simulink model "MEAS_Speed_Read"  (R2022b)
settings: Solver=FixedStepDiscrete  StartTime=0.0  StopTime=10.0  RelTol=1e-3  EnableMultiTasking=on
InitFcn:
  | mbd_mpc_consistency_checks(bdroot(gcs));
undefined symbols (not defined in the file): AngleChangeDir, I_MAX, LQFP, OffsetSelector, PhA_Offset, PhB_Offset, SpdChangeDir, SpdFilterConst
libraries: mbd_mpc574x_ec_toolbox x18, ammclib_bam_mpc574x x9, simulink x1, mcbpositiondecoderlib x1
settings Model: Creator=MAAM  LastModifiedBy=MAAM
settings DataIOCC: ExternalInput=off  InitialState=off  SaveOutput=off  SignalLogging=off  SaveTime=off
settings OptimizationCC: DefaultParameterBehavior=Inlined  EnhancedBackFolding=on  PassReuseOutputArgsAs=Individual arguments  ZeroExternalMemoryAtStartup=off  ZeroInternalMemoryAtStartup=off  OptimizeBlockOrder=speed  DifferentSizesBufferReuse=on  OptimizationCustomize=off  EfficientTunableParamExpr=on
settings DebuggingCC: InheritedTsInSrcMsg=none  ParameterTunabilityLossMsg=error
settings HardwareCC: ProdBitPerPointer=32  ProdBitPerSizeT=32  ProdBitPerPtrDiffT=32  ProdLargestAtomicInteger=Long  ProdLargestAtomicFloat=Double  ProdEndianess=BigEndian  ProdWordSize=32  ProdHWDeviceType=Motorola PowerPC
settings ModelReferenceCC: ModelReferenceNumInstancesAllowed=Single
settings SFSimCC: MATLABDynamicMemAlloc=off
settings RTWCC: Description=Model Based Design Toolbox MPC57xx Code Generation Target  SystemTargetFile=mbd_mpc574x.tlc  MakeCommand=mbd_mpc574x_make_rtw  TemplateMakefile=mbd_mpc574x.tmf
settings CodeAppCC: ForceParamTrailComments=on  IgnoreCustomStorageClasses=off  OperatorAnnotations=on  SimulinkDataObjDesc=on  SFDataObjDesc=on  InsertBlockDesc=on
settings STFCustomTargetCC: TargetLangStandard=C99 (ISO)  MultiwordLength=256  CombineOutputUpdateFcns=on  ERTCustomFileBanners=on  SupportContinuousTime=off  SupportNonInlinedSFcns=off  RemoveResetFunc=on  MATLABClassNameForMDSCustomization=Simulink.SoftwareTarget.ERTCustomization  SystemTargetFile=mbd_mpc574x.tlc
settings ERTTargetCC: TargetLangStandard=C99 (ISO)  ParMdlRefBuildCompliant=off  CompOptLevelCompliant=off  ConcurrentExecutionCompliant=off  ModelStepFunctionPrototypeControlCompliant=off  CPPClassGenCompliant=off  UseToolchainInfoCompliant=off  InlinedParameterPlacement=NonHierarchical  ERTCustomFileTemplate=example_file_process.tlc

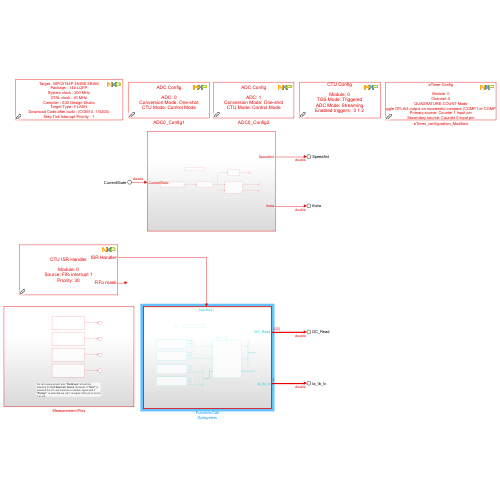
[thumbnail: Simulink's stored preview of the top-level diagram]
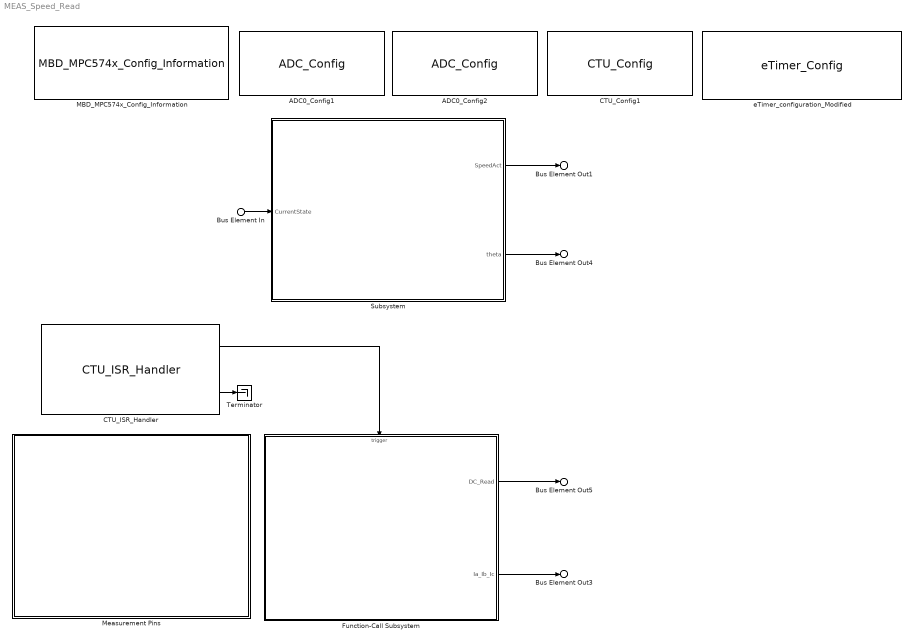
== system MEAS_Speed_Read ==
  Bus Element In : Inport  PortName=CurrentState
  ADC0_Config1 : mbd_mpc574x_ec_toolbox/Motor Control Blocks/ADC Blocks/ADC_Config  Priority=9  adc_instance=0  adc_mode=One-shot  adc_ctu=Control Mode  adc_channels_no_n=3  adc_channel_n_0=PTB9: [ADC0_AN11 | Analog function AN11 of ADC0]  adc_channel_n_1=PTB12: [ADC0_AN14 | Analog function AN14 of ADC0]  adc_channel_n_2=PTB8: [ADC0_AN1 | Analog function AN1 of ADC0]  adc_channel_n_3=not available  adc_channel_n_4=not available  adc_channel_n_5=not available  adc_channel_n_6=not available  adc_channel_n_7=not available  adc_channel_n_8=not available  adc_channel_n_9=not available  adc_channel_n_10=not available  adc_channel_n_11=not available  adc_channel_n_12=not available  adc_channel_n_13=not available  adc_channel_n_14=not available  adc_channel_n_15=not available  adc_channel_n_16=not available  adc_channel_n_17=not available  adc_channel_n_18=not available  adc_channel_n_19=not available  adc_channel_n_20=not available  adc_channel_n_21=not available  adc_channel_n_22=not available  adc_channel_n_23=not available  adc_channel_n_24=not available  adc_channel_n_25=not available  adc_channel_n_26=not available  adc_channel_n_27=not available  adc_channel_n_28=not available  adc_channel_n_29=not available  adc_channel_n_30=not available  adc_channel_n_31=not available  adc_channel_n_32=not available  adc_channel_n_33=not available  adc_channel_n_34=not available  adc_channel_n_35=not available  adc_channel_n_36=not available  adc_channel_n_37=not available  adc_channel_n_38=not available  adc_channel_n_39=not available  adc_channel_n_40=not available  adc_channel_n_41=not available  adc_channel_n_42=not available  adc_channel_n_43=not available  adc_channel_n_44=not available  adc_channel_n_45=not available  adc_channel_n_46=not available  adc_channel_n_47=not available  show_adv_opts=on  adc_prec=8  adc_presample_0=High voltage ground for ADC  adc_int=8  adc_presample_1=High voltage ground for ADC  adc_ext=8  adc_presample_2=High voltage ground for ADC  adc_clk=Equal to bus clock  adc_ack=off  adc_ext_trigger=External Trigger Disabled  adc_skip_sampling=off  adc_calibration=on  adc_wls=Right  adc_owr=off  adc_inj_trigger=Injected Trigger Disabled  adc_mux_delay=0  adc_decode_delay=0  adc_thr_reg_no=0  adc_upper_value_0=0  adc_lower_value_0=0  adc_upper_value_1=0  adc_lower_value_1=0  adc_upper_value_2=0  adc_lower_value_2=0  adc_upper_value_3=0  adc_lower_value_3=0  adc_upper_value_4=0  adc_lower_value_4=0  adc_upper_value_5=0  adc_lower_value_5=0  adc_upper_value_6=0  adc_lower_value_6=0  adc_upper_value_7=0  adc_lower_value_7=0  adc_upper_value_8=0  adc_lower_value_8=0  adc_upper_value_9=0  adc_lower_value_9=0  adc_upper_value_10=0  adc_lower_value_10=0  adc_upper_value_11=0  adc_lower_value_11=0  adc_upper_value_12=0  adc_lower_value_12=0  adc_upper_value_13=0  adc_lower_value_13=0  adc_upper_value_14=0  adc_lower_value_14=0  adc_upper_value_15=0  adc_lower_value_15=0  adc_wdt_isr_init=off  adc_en_wdt_0=off  adc_th_index_0=0  adc_en_wdt_1=off  adc_th_index_1=0  adc_en_wdt_2=off  adc_th_index_2=0  adc_en_wdt_3=off  adc_th_index_3=0  adc_en_wdt_4=off  adc_th_index_4=0  adc_en_wdt_5=off  adc_th_index_5=0  adc_en_wdt_6=off  adc_th_index_6=0  adc_en_wdt_7=off  adc_th_index_7=0  adc_en_wdt_8=off  adc_th_index_8=0  adc_en_wdt_9=off  adc_th_index_9=0  adc_en_wdt_10=off  adc_th_index_10=0  adc_en_wdt_11=off  adc_th_index_11=0  adc_en_wdt_12=off  adc_th_index_12=0  adc_en_wdt_13=off  adc_th_index_13=0  adc_en_wdt_14=off  adc_th_index_14=0  adc_en_wdt_15=off  adc_th_index_15=0  adc_en_wdt_16=off  adc_th_index_16=0  adc_en_wdt_17=off  adc_th_index_17=0  adc_en_wdt_18=off  adc_th_index_18=0  adc_en_wdt_19=off  adc_th_index_19=0  adc_en_wdt_20=off  adc_th_index_20=0  adc_en_wdt_21=off  adc_th_index_21=0  adc_en_wdt_22=off  adc_th_index_22=0  adc_en_wdt_23=off  adc_th_index_23=0  adc_en_wdt_24=off  adc_th_index_24=0  adc_en_wdt_25=off  adc_th_index_25=0  adc_en_wdt_26=off  adc_th_index_26=0  adc_en_wdt_27=off  adc_th_index_27=0  adc_en_wdt_28=off  adc_th_index_28=0  adc_en_wdt_29=off  adc_th_index_29=0  adc_en_wdt_30=off  adc_th_index_30=0  adc_en_wdt_31=off  adc_th_index_31=0  adc_en_wdt_32=off  adc_th_index_32=0  adc_en_wdt_33=off  adc_th_index_33=0  adc_en_wdt_34=off  adc_th_index_34=0  adc_en_wdt_35=off  adc_th_index_35=0  adc_en_wdt_36=off  adc_th_index_36=0  adc_en_wdt_37=off  adc_th_index_37=0  adc_en_wdt_38=off  adc_th_index_38=0  adc_en_wdt_39=off  adc_th_index_39=0  adc_en_wdt_40=off  adc_th_index_40=0  adc_en_wdt_41=off  adc_th_index_41=0  adc_en_wdt_42=off  adc_th_index_42=0  adc_en_wdt_43=off  adc_th_index_43=0  adc_en_wdt_44=off  adc_th_index_44=0  adc_en_wdt_45=off  adc_th_index_45=0  adc_en_wdt_46=off  adc_th_index_46=0  adc_en_wdt_47=off  adc_th_index_47=0
  ADC0_Config2 : mbd_mpc574x_ec_toolbox/Motor Control Blocks/ADC Blocks/ADC_Config  Priority=9  adc_instance=1  adc_mode=One-shot  adc_ctu=Control Mode  adc_channels_no_n=1  adc_channel_n_0=PTB10: [ADC1_AN12 | Analog function AN12 of ADC1]  adc_channel_n_1=not available  adc_channel_n_2=not available  adc_channel_n_3=not available  adc_channel_n_4=not available  adc_channel_n_5=not available  adc_channel_n_6=not available  adc_channel_n_7=not available  adc_channel_n_8=not available  adc_channel_n_9=not available  adc_channel_n_10=not available  adc_channel_n_11=not available  adc_channel_n_12=not available  adc_channel_n_13=not available  adc_channel_n_14=not available  adc_channel_n_15=not available  adc_channel_n_16=not available  adc_channel_n_17=not available  adc_channel_n_18=not available  adc_channel_n_19=not available  adc_channel_n_20=not available  adc_channel_n_21=not available  adc_channel_n_22=not available  adc_channel_n_23=not available  adc_channel_n_24=not available  adc_channel_n_25=not available  adc_channel_n_26=not available  adc_channel_n_27=not available  adc_channel_n_28=not available  adc_channel_n_29=not available  adc_channel_n_30=not available  adc_channel_n_31=not available  adc_channel_n_32=not available  adc_channel_n_33=not available  adc_channel_n_34=not available  adc_channel_n_35=not available  adc_channel_n_36=not available  adc_channel_n_37=not available  adc_channel_n_38=not available  adc_channel_n_39=not available  adc_channel_n_40=not available  adc_channel_n_41=not available  adc_channel_n_42=not available  adc_channel_n_43=not available  adc_channel_n_44=not available  adc_channel_n_45=not available  adc_channel_n_46=not available  adc_channel_n_47=not available  show_adv_opts=on  adc_prec=8  adc_presample_0=High voltage ground for ADC  adc_int=8  adc_presample_1=High voltage ground for ADC  adc_ext=8  adc_presample_2=High voltage ground for ADC  adc_clk=Equal to bus clock  adc_ack=off  adc_ext_trigger=External Trigger Disabled  adc_skip_sampling=off  adc_calibration=on  adc_wls=Right  adc_owr=off  adc_inj_trigger=Injected Trigger Disabled  adc_mux_delay=0  adc_decode_delay=0  adc_thr_reg_no=0  adc_upper_value_0=0  adc_lower_value_0=0  adc_upper_value_1=0  adc_lower_value_1=0  adc_upper_value_2=0  adc_lower_value_2=0  adc_upper_value_3=0  adc_lower_value_3=0  adc_upper_value_4=0  adc_lower_value_4=0  adc_upper_value_5=0  adc_lower_value_5=0  adc_upper_value_6=0  adc_lower_value_6=0  adc_upper_value_7=0  adc_lower_value_7=0  adc_upper_value_8=0  adc_lower_value_8=0  adc_upper_value_9=0  adc_lower_value_9=0  adc_upper_value_10=0  adc_lower_value_10=0  adc_upper_value_11=0  adc_lower_value_11=0  adc_upper_value_12=0  adc_lower_value_12=0  adc_upper_value_13=0  adc_lower_value_13=0  adc_upper_value_14=0  adc_lower_value_14=0  adc_upper_value_15=0  adc_lower_value_15=0  adc_wdt_isr_init=off  adc_en_wdt_0=off  adc_th_index_0=0  adc_en_wdt_1=off  adc_th_index_1=0  adc_en_wdt_2=off  adc_th_index_2=0  adc_en_wdt_3=off  adc_th_index_3=0  adc_en_wdt_4=off  adc_th_index_4=0  adc_en_wdt_5=off  adc_th_index_5=0  adc_en_wdt_6=off  adc_th_index_6=0  adc_en_wdt_7=off  adc_th_index_7=0  adc_en_wdt_8=off  adc_th_index_8=0  adc_en_wdt_9=off  adc_th_index_9=0  adc_en_wdt_10=off  adc_th_index_10=0  adc_en_wdt_11=off  adc_th_index_11=0  adc_en_wdt_12=off  adc_th_index_12=0  adc_en_wdt_13=off  adc_th_index_13=0  adc_en_wdt_14=off  adc_th_index_14=0  adc_en_wdt_15=off  adc_th_index_15=0  adc_en_wdt_16=off  adc_th_index_16=0  adc_en_wdt_17=off  adc_th_index_17=0  adc_en_wdt_18=off  adc_th_index_18=0  adc_en_wdt_19=off  adc_th_index_19=0  adc_en_wdt_20=off  adc_th_index_20=0  adc_en_wdt_21=off  adc_th_index_21=0  adc_en_wdt_22=off  adc_th_index_22=0  adc_en_wdt_23=off  adc_th_index_23=0  adc_en_wdt_24=off  adc_th_index_24=0  adc_en_wdt_25=off  adc_th_index_25=0  adc_en_wdt_26=off  adc_th_index_26=0  adc_en_wdt_27=off  adc_th_index_27=0  adc_en_wdt_28=off  adc_th_index_28=0  adc_en_wdt_29=off  adc_th_index_29=0  adc_en_wdt_30=off  adc_th_index_30=0  adc_en_wdt_31=off  adc_th_index_31=0  adc_en_wdt_32=off  adc_th_index_32=0  adc_en_wdt_33=off  adc_th_index_33=0  adc_en_wdt_34=off  adc_th_index_34=0  adc_en_wdt_35=off  adc_th_index_35=0  adc_en_wdt_36=off  adc_th_index_36=0  adc_en_wdt_37=off  adc_th_index_37=0  adc_en_wdt_38=off  adc_th_index_38=0  adc_en_wdt_39=off  adc_th_index_39=0  adc_en_wdt_40=off  adc_th_index_40=0  adc_en_wdt_41=off  adc_th_index_41=0  adc_en_wdt_42=off  adc_th_index_42=0  adc_en_wdt_43=off  adc_th_index_43=0  adc_en_wdt_44=off  adc_th_index_44=0  adc_en_wdt_45=off  adc_th_index_45=0  adc_en_wdt_46=off  adc_th_index_46=0  adc_en_wdt_47=off  adc_th_index_47=0
  CTU_Config1 : mbd_mpc574x_ec_toolbox/Motor Control Blocks/CTU Blocks/CTU_Config  Priority=10  ctuModule=0  ctuPrescaler=1  ctuTGS=Triggered  ctuTGSCCV=7000  ctuTGSCLM=0  ctuExtMode=Toggle  ctuTGSADC=Streaming  ctuMrsInput=PWM Reload  ctuMrsInputEdge=Rising Edge  ctuMrsIsrEnable=off  ctuIsrErrEnable=off  ctuDMAGREEnable=off  ctuMRSDMAEnable=off  ctuDisableoutput=off  ctuShowAdvOpts=on  inputPwmRel=Rising Edge  inputPwmOdd0=Disabled  inputPwmOdd1=Disabled  inputPwmOdd2=Disabled  inputPwmOdd3=Disabled  inputPwmEven0=Disabled  inputPwmEven1=Disabled  inputPwmEven3=Disabled  inputPwmEven2=Disabled  inputPwmReal0=Disabled  inputPwmReal1=Disabled  inputPwmReal2=Disabled  inputPwmReal3=Disabled  inputeTimer1=Disabled  inputeTimer2=Disabled  inputExternal=Disabled  trgEn0=on  trgEn1=on  trgEn2=on  trgEn3=off  trgEn4=off  trgEn5=off  trgEn6=off  trgEn7=off  trgCmp0=250  trgExt0=off  trgTmr0_0=off  trgTmr1_0=off  trgTmr2_0=off  trgInt0=off  trgAdc0=on  trgAdcStart0=0  trgAdcStop0=0  trgCmp1=1000  trgExt1=off  trgTmr0_1=off  trgTmr1_1=off  trgTmr2_1=off  trgInt1=off  trgAdc1=on  trgAdcStart1=1  trgAdcStop1=1  trgCmp2=0  trgExt2=off  trgTmr0_2=off  trgTmr1_2=off  trgTmr2_2=off  trgInt2=off  trgAdc2=on  trgAdcStart2=2  trgAdcStop2=2  trgCmp3=0  trgExt3=off  trgTmr0_3=off  trgTmr1_3=off  trgTmr2_3=off  trgInt3=off  trgAdc3=off  trgAdcStart3=0  trgAdcStop3=0  trgCmp4=0  trgExt4=off  trgTmr0_4=off  trgTmr1_4=off  trgTmr2_4=off  trgInt4=off  trgAdc4=off  trgAdcStart4=0  trgAdcStop4=0  trgCmp5=0  trgExt5=off  trgTmr0_5=off  trgTmr1_5=off  trgTmr2_5=off  trgAdc5=off  trgInt5=off  trgAdcStart5=0  trgAdcStop5=0  trgCmp6=0  trgExt6=off  trgTmr0_6=off  trgTmr1_6=off  trgTmr2_6=off  trgInt6=off  trgAdc6=off  trgAdcStart6=0  trgAdcStop6=0  trgCmp7=0  trgExt7=off  trgTmr0_7=off  trgTmr1_7=off  trgTmr2_7=off  trgInt7=off  trgAdc7=off  trgAdcStart7=0  trgAdcStop7=0  fifoTh0=1  fifoIsrOVR0=off  fifoIsrOVF0=off  fifoIsrEmpty0=off  fifoIsrFull0=off  fifoDMA0=off  fifoTh1=3  fifoIsrOVR1=off  fifoIsrOVF1=on  fifoIsrEmpty1=off  fifoIsrFull1=off  fifoDMA1=off  fifoTh2=0  fifoIsrOVR2=off  fifoIsrOVF2=off  fifoIsrEmpty2=off  fifoIsrFull2=off  fifoDMA2=off  fifoTh3=0  fifoIsrOVR3=off  fifoIsrOVF3=off  fifoIsrEmpty3=off  fifoIsrFull3=off  fifoDMA3=off  pinInternal=None  pinExternal=PTC14: [CTU0_EXT_TGR | CTU0 External Trigger Output]  ctuAdcCmdNumber=3  adc_ie_0=off  adc_fifo_0=1  adc_conv_mode_0=Single Conversion  adc_port_0=Port A  adc_channel_0=14  adc_channel_a_0=0  adc_channel_b_0=0  adc_ie_1=off  adc_fifo_1=1  adc_conv_mode_1=Single Conversion  adc_port_1=Port A  adc_channel_1=1  adc_channel_a_1=0  adc_channel_b_1=0  adc_ie_2=off  adc_fifo_2=1  adc_conv_mode_2=Dual Conversion  adc_port_2=Port A  adc_channel_2=11  adc_channel_a_2=11  adc_channel_b_2=12  adc_ie_3=off  adc_fifo_3=1  adc_conv_mode_3=Single Conversion  adc_port_3=Port B  adc_channel_3=12  adc_channel_a_3=0  adc_channel_b_3=0  adc_ie_4=off  adc_fifo_4=0  adc_conv_mode_4=Single Conversion  adc_port_4=Port A  adc_channel_4=0  adc_channel_a_4=0  adc_channel_b_4=0  adc_ie_5=off  adc_fifo_5=0  adc_conv_mode_5=Single Conversion  adc_port_5=Port A  adc_channel_5=0  adc_channel_a_5=0  adc_channel_b_5=0  adc_ie_6=off  adc_fifo_6=0  adc_conv_mode_6=Single Conversion  adc_port_6=Port A  adc_channel_6=0  adc_channel_a_6=0  adc_channel_b_6=0  adc_ie_7=off  adc_fifo_7=0  adc_conv_mode_7=Single Conversion  adc_port_7=Port A  adc_channel_7=0  adc_channel_a_7=0  adc_channel_b_7=0  adc_ie_8=off  adc_fifo_8=0  adc_conv_mode_8=Single Conversion  adc_port_8=Port A  adc_channel_8=0  adc_channel_a_8=0  adc_channel_b_8=0  adc_ie_9=off  adc_fifo_9=0  adc_conv_mode_9=Single Conversion  adc_port_9=Port A  adc_channel_9=0  adc_channel_a_9=0  adc_channel_b_9=0  adc_ie_10=off  adc_fifo_10=0  adc_conv_mode_10=Single Conversion  adc_port_10=Port A  adc_channel_10=0  adc_channel_a_10=0  adc_channel_b_10=0  adc_ie_11=off  adc_fifo_11=0  adc_conv_mode_11=Single Conversion  adc_port_11=Port A  adc_channel_11=0  adc_channel_a_11=0  adc_channel_b_11=0  adc_ie_12=off  adc_fifo_12=1  adc_conv_mode_12=Single Conversion  adc_port_12=Port A  adc_channel_12=0  adc_channel_a_12=0  adc_channel_b_12=0  adc_ie_13=off  adc_fifo_13=3  adc_conv_mode_13=Single Conversion  adc_port_13=Port A  adc_channel_13=0  adc_channel_a_13=0  adc_channel_b_13=0  adc_ie_14=off  adc_fifo_14=0  adc_conv_mode_14=Single Conversion  adc_port_14=Port A  adc_channel_14=0  adc_channel_a_14=0  adc_channel_b_14=0  adc_ie_15=off  adc_fifo_15=0  adc_conv_mode_15=Single Conversion  adc_port_15=Port A  adc_channel_15=0  adc_channel_a_15=0  adc_channel_b_15=0  adc_ie_16=off  adc_fifo_16=0  adc_conv_mode_16=Single Conversion  adc_port_16=Port A  adc_channel_16=0  adc_channel_a_16=0  adc_channel_b_16=0  adc_ie_17=off  adc_fifo_17=0  adc_conv_mode_17=Single Conversion  adc_port_17=Port A  adc_channel_17=0  adc_channel_a_17=0  adc_channel_b_17=0  adc_ie_18=off  adc_fifo_18=0  adc_conv_mode_18=Single Conversion  adc_port_18=Port A  adc_channel_18=0  adc_channel_a_18=0  adc_channel_b_18=0  adc_ie_19=off  adc_fifo_19=0  adc_conv_mode_19=Single Conversion  adc_port_19=Port A  adc_channel_19=0  adc_channel_a_19=0  adc_channel_b_19=0  adc_ie_20=off  adc_fifo_20=0  adc_conv_mode_20=Single Conversion  adc_port_20=Port A  adc_channel_20=0  adc_channel_a_20=0  adc_channel_b_20=0  adc_ie_21=off  adc_fifo_21=0  adc_conv_mode_21=Single Conversion  adc_port_21=Port A  adc_channel_21=0  adc_channel_a_21=0  adc_channel_b_21=0  adc_ie_22=off  adc_fifo_22=0  adc_conv_mode_22=Single Conversion  adc_port_22=Port A  adc_channel_22=0  adc_channel_a_22=0  adc_channel_b_22=0  adc_ie_23=off  adc_fifo_23=0  adc_conv_mode_23=Single Conversion  adc_port_23=Port A  adc_channel_23=0  adc_channel_a_23=0  adc_channel_b_23=0
  CTU_ISR_Handler : mbd_mpc574x_ec_toolbox/Motor Control Blocks/CTU Blocks/CTU_ISR_Handler  ctuModule=0  ctuIsrSource=Fifo interrupt  ctuIsrPriority=30  ctuIsrTrigger=1  ctuIsrFifo=1
  Function-Call Subsystem : Subsystem  TreatAsAtomicUnit=on
  MBD_MPC574x_Config_Information : mbd_mpc574x_ec_toolbox/MBD_MPC574x_Config_Information  Priority=1  disp_str=|  config_params=[]  mcu_target_name=MPC5744P  mcu_target_package=144-LQFP  mcu_target_sram_size=384KB  mcu_system_clock_freq=200  mcu_xtal_freq=40  mcu_step_timer=PIT Channel 0  mcu_step_priority=1  ds_import_enable=on  target_compiler=S32 Design Studio  target_memory=FLASH  s32ds_target_compile_opts=-g3 -mbig -mvle -O1 -mregnames -mlsp -specs=ewl_c9x.specs -mhard-float -Wall -c -std=c99 -fdata-sections -ffunction-sections -funsigned-char -fmessage-length=0 -nostdinc -fno-jump-tables -DTURN_ON_CPU0  s32ds_target_assemble_opts=-g3 -mbig -mvle -mregnames -O1 -DTURN_ON_CPU0 -mhard-float  s32ds_target_link_opts=-Xlinker -gc-sections  s32ds_target_default_lcf=on  s32ds_target_user_lcf=MPC5744P_flash.ld  ghs_target_compile_opts=-G -filetype.c  ghs_target_assemble_opts=-G -filetype.assembly  ghs_target_default_lcf=on  ghs_target_user_lcf=MPC5744P_flash.ld  diab_target_compile_opts=-@E+err.log -c -g -Xenum-is-best -Xlint -Xnested-interrupts -Xdebug-local-cie -Xclib-optim-off -Xc-new  diab_target_assemble_opts=-@E+err.log -l -g  diab_target_link_opts=-@E+err.log -Ws -m6 -lc -lm  diab_target_default_lcf=on  diab_target_user_lcf=MPC5744P_flash.dld  pil_download_enable=off  rbl_download_enable=on  rbl_start_delay=5000  rbl_restart_request=on  rbl_com_port=Custom  rbl_com_port_custom=COM10  pil_download_rate=115200  pil_interface=Serial 0  pil_rx=PTB3: [LIN0_RX | LIN 0 Receive Pin]  pil_tx=PTB2: [LIN0_TX | LINFlexD 0 Transmit Pin]  rbl_def_password=on  rbl_password=0xFEEDFACECAFEBEEF  rbl_manual_len_size=off  rbl_start_address=0  rbl_code_size=0  ADC_PcrCheckEnDis=on  FlexPWM_PcrCheckEnDis=on  CTU_PcrCheckEnDis=on  SWG_PcrCheckEnDis=on  eTimer_PcrCheckEnDis=off  EQADC_PcrCheckEnDis=on  eMIOS_PcrCheckEnDis=on  FlexCAN_PcrCheckEnDis=on  I2C_PcrCheckEnDis=on  MCAN_PcrCheckEnDis=on  SPI_PcrCheckEnDis=on  UART_PcrCheckEnDis=on  GPIO_OutputPcrCheckEnDis=on  GPIO_InputPcrCheckEnDis=on  eDMA_PcrCheckEnDis=on  PIT_PcrCheckEnDis=on  AMMCLIB_PcrCheckEnDis=on  FM_PcrCheckEnDis=on  Profiler_PcrCheckEnDis=on  ModelRef_PcrCheckEnDis=on  ModelPinCheck_PcrCheckEnDis=on
      | System Clock : 200 MHz
      | Target : MPC5744P
      | Package : 144LQFP
      | XTAL Freq : 40 MHz
      | Compiler : S32 Design Studio
      | Target Type : FLASH
      | Global Interrupt Priority : 8
      | System Tick Interrupt Priority : 12
      | Freemaster : None;
      | Download Code after build : off
  Measurement Pins : Subsystem
  Subsystem : Subsystem
  Terminator : Terminator
  eTimer_configuration_Modified : mbd_mpc574x_ec_toolbox/Motor Control Blocks/eTIMER Blocks/eTimer_Config  etimerModule=0  etimerChannel=0  etimerMode=QUADRATURE-COUNT Mode  etimerCountOnce=Count repeatedly  etimerCountLength=Count until compare and then reinitialize  etimerCountDirection=Count down  etimerCountStart=on  etimerCaptureArm=on  etimerShowAdv=on  etimerPrimarySource=Counter 1 input pin  etimerPrimaryPolarity=True polarity  etimerSecondarySource=Counter 0 input pin  etimerSecondaryPolarity=True polarity  etimerSampleCount=Require 3 consecutive samples to be of equal value  etimerSamplePeriod=1  etimerOutEnable=The external pin is configured as an input  etimerOutPolarity=True polarity  etimerOutMode=Toggle OFLAG output on successful compare (COMP1 or COMP2)  etimerCompMode=COMP1 is used when the counter is counting up and COMP2 when counting down  etimerCompLoad1=Load CNTR with CMPLD upon successful compare with the value in COMP2  etimerCompLoad2=Load CNTR with CMPLD upon successful compare with the value in COMP1  etimerCapt1=Capture any edge  etimerCapt2=Capture any edge  etimerOneShot=Free running mode is selected  etimerMasterMode=Disable broadcast of this channel output  etimerCoForce=Other channels cannot force this channel output  etimerCoChanInit=Other channels cannot force re-initialization of this channel  etimerRedundant=off  etimerCOMP1init=3999  etimerCOMP2init=0  etimerCNTRinit=0  etimerCh0=PTA0: [eTimer0_ETC0 | eTimer_0 Input Data Channel 0]  etimerCh1=PTA1: [eTimer0_ETC1 | eTimer_0 Input Data Channel 1]  etimerCh2=None  etimerCh3=None  etimerCh4=None  etimerCh5=None  etimerIsrTCFIE=off  etimerIsrTCF1IE=off  etimerIsrTCF2IE=off  etimerIsrTOFIE=off  etimerIsrIELFIE=off  etimerIsrIEHFIE=off  etimerIsrICF1IE=off  etimerIsrICF2IE=off  etimerIsrRCF=off  etimerIsrWDF=off
  Bus Element Out1 : Outport  PortName=SpeedAct
  Bus Element Out3 : Outport  Port=2  PortName=Ia_Ib_Ic
  Bus Element Out4 : Outport  Port=3  PortName=theta
  Bus Element Out5 : Outport  Port=4  PortName=DC_Read
  wires:
  Subsystem/1(SpeedAct) -> Bus Element Out1/1
  CTU_ISR_Handler/2 -> Terminator/1
  CTU_ISR_Handler/1 -> Function-Call Subsystem/Trigger
  Function-Call Subsystem/2(Ia_Ib_Ic) -> Bus Element Out3/1
  Subsystem/2(theta) -> Bus Element Out4/1
  Function-Call Subsystem/1(DC_Read) -> Bus Element Out5/1
  Bus Element In/1 -> Subsystem/1(CurrentState)

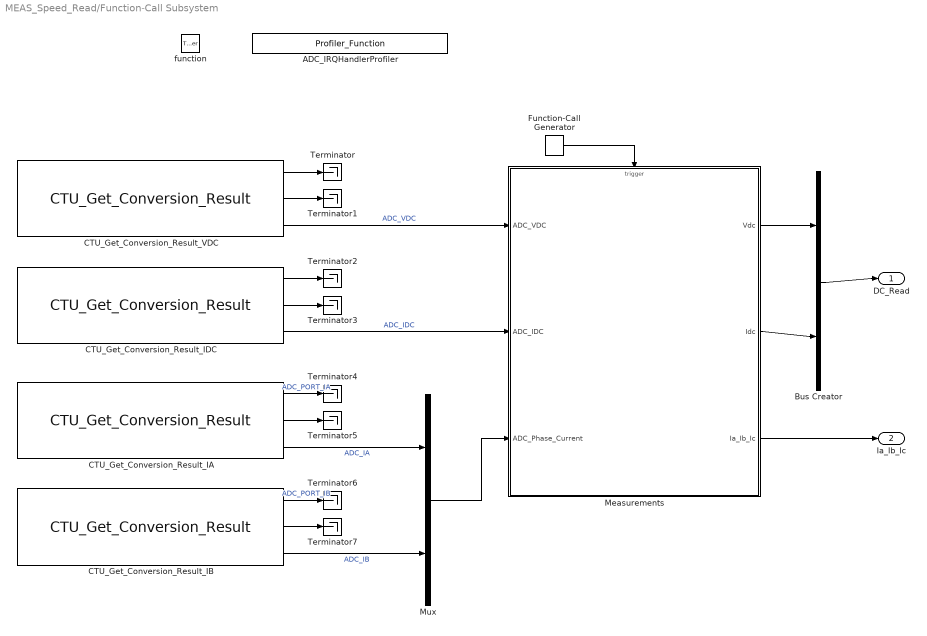
== system MEAS_Speed_Read/Function-Call Subsystem ==
  function : TriggerPort  TriggerType=function-call  VariantControl=(inherit)
  ADC_IRQHandlerProfiler : mbd_mpc574x_ec_toolbox/Utility Blocks/Profiler_Function  profile_index=2
  Bus Creator : BusCreator  Inputs=2
  CTU_Get_Conversion_Result_IA : mbd_mpc574x_ec_toolbox/Motor Control Blocks/CTU Blocks/CTU_Get_Conversion_Result  Priority=3  ctuModule=0  ctuFifoIndex=1  ctuAlign=Right unsigned
  CTU_Get_Conversion_Result_IB : mbd_mpc574x_ec_toolbox/Motor Control Blocks/CTU Blocks/CTU_Get_Conversion_Result  Priority=4  ctuModule=0  ctuFifoIndex=1  ctuAlign=Right unsigned
  CTU_Get_Conversion_Result_IDC : mbd_mpc574x_ec_toolbox/Motor Control Blocks/CTU Blocks/CTU_Get_Conversion_Result  Priority=2  ctuModule=0  ctuFifoIndex=1  ctuAlign=Right unsigned
  CTU_Get_Conversion_Result_VDC : mbd_mpc574x_ec_toolbox/Motor Control Blocks/CTU Blocks/CTU_Get_Conversion_Result  Priority=1  ctuModule=0  ctuFifoIndex=1  ctuAlign=Right unsigned
  Function-Call Generator : simulink/Ports & Subsystems/Function-Call Generator  sample_time=-1  numberOfIterations=1  DisallowWideOutput=off
  Measurements : Subsystem  TreatAsAtomicUnit=on
  Mux : Mux  Inputs=2
  Terminator{,1..7} (8 alike) : Terminator
  DC_Read : Outport
  Ia_Ib_Ic : Outport  Port=2
  wires:
  CTU_Get_Conversion_Result_IB/2 -> Terminator7/1
  CTU_Get_Conversion_Result_IB/1 -> Terminator6/1  "ADC_PORT_IB"
  CTU_Get_Conversion_Result_IA/2 -> Terminator5/1
  CTU_Get_Conversion_Result_IA/1 -> Terminator4/1  "ADC_PORT_IA"
  CTU_Get_Conversion_Result_IDC/2 -> Terminator3/1
  CTU_Get_Conversion_Result_IDC/1 -> Terminator2/1
  CTU_Get_Conversion_Result_VDC/2 -> Terminator1/1
  CTU_Get_Conversion_Result_VDC/1 -> Terminator/1
  CTU_Get_Conversion_Result_IB/3 -> Mux/2  "ADC_IB"
  CTU_Get_Conversion_Result_IA/3 -> Mux/1  "ADC_IA"
  Mux/1 -> Measurements/3(ADC_Phase_Current)
  Function-Call Generator/1 -> Measurements/Trigger
  CTU_Get_Conversion_Result_IDC/3 -> Measurements/2(ADC_IDC)  "ADC_IDC"
  CTU_Get_Conversion_Result_VDC/3 -> Measurements/1(ADC_VDC)  "ADC_VDC"
  Measurements/1(Vdc) -> Bus Creator/1
  Measurements/2(Idc) -> Bus Creator/2
  Measurements/3(Ia_Ib_Ic) -> Ia_Ib_Ic/1
  Bus Creator/1 -> DC_Read/1

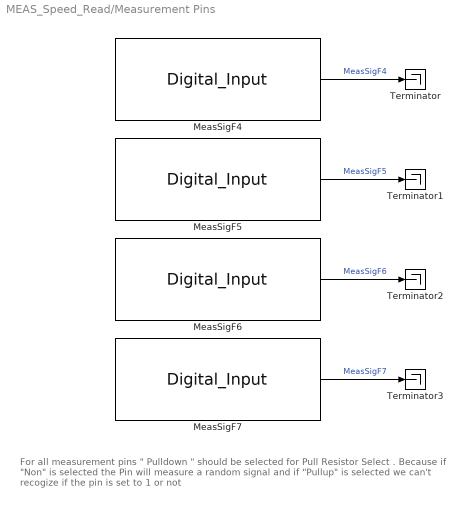
== system MEAS_Speed_Read/Measurement Pins ==
  note: For all measurement pins " Pulldown " should be selected for Pull Resistor Select . Because if "Non" is selected the Pin will measure a random signal and if "Pullup" is selected we can't recogize if the pin is set to 1 or not
  MeasSigF4 : mbd_mpc574x_ec_toolbox/GPIO Blocks/Digital_Input  gpio_pin=PTF4: [SIUL2_GPIO84 | General Purpose IO PF[4]]  pull_resistor=Pulldown
  MeasSigF5 : mbd_mpc574x_ec_toolbox/GPIO Blocks/Digital_Input  gpio_pin=PTF5: [SIUL2_GPIO85 | General Purpose IO PF[5]]  pull_resistor=Pulldown
  MeasSigF6 : mbd_mpc574x_ec_toolbox/GPIO Blocks/Digital_Input  gpio_pin=PTF6: [SIUL2_GPIO86 | General Purpose IO PF[6]]  pull_resistor=Pulldown
  MeasSigF7 : mbd_mpc574x_ec_toolbox/GPIO Blocks/Digital_Input  gpio_pin=PTE7: [SIUL2_GPI71 | General Purpose IO PE[7]]  pull_resistor=Pulldown
  Terminator{,1..3} (4 alike) : Terminator
  wires:
  MeasSigF5/1 -> Terminator1/1  "MeasSigF5"
  MeasSigF4/1 -> Terminator/1  "MeasSigF4"
  MeasSigF7/1 -> Terminator3/1  "MeasSigF7"
  MeasSigF6/1 -> Terminator2/1  "MeasSigF6"

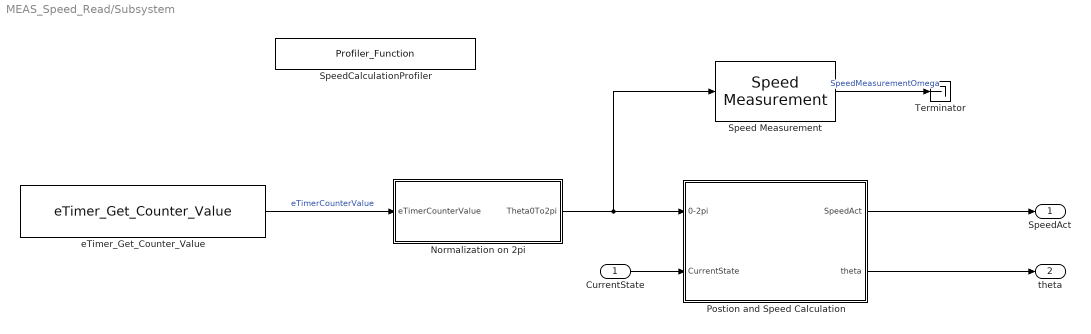
== system MEAS_Speed_Read/Subsystem ==
  CurrentState : Inport
  Normalization on 2pi : Subsystem
  Postion and Speed Calculation : Subsystem
  Speed Measurement : mcbpositiondecoderlib/Speed Measurement  PositionUnit=Radians  PositionScalingDatatype=uint32  SpeedCalculationMode=Maximum application speed  SampleTimeAsync=100e-6  MaximumApplicationSpeed=3000  SpeedResolution=5e-6  DelayLength=99  MaximumMeasurableSpeed=3000  MeasurableSpeedResolution=1.397e-06  SpeedUnit=RPM  PerUnitSpeed=1000  SpeedDataType=single
  "SpeedCalculationProfiler   " : mbd_mpc574x_ec_toolbox/Utility Blocks/Profiler_Function  profile_index=4
  Terminator : Terminator
  eTimer_Get_Counter_Value : mbd_mpc574x_ec_toolbox/Motor Control Blocks/eTIMER Blocks/eTimer_Get_Counter_Value  etimerModule=0  etimerChannel=0
  SpeedAct : Outport
  theta : Outport  Port=2
  wires:
  Normalization on 2pi/1(Theta0To2pi) -> Speed Measurement/1, Postion and Speed Calculation/1(0-2pi)
  Speed Measurement/1 -> Terminator/1  "SpeedMeasurementOmega"
  eTimer_Get_Counter_Value/1 -> Normalization on 2pi/1(eTimerCounterValue)  "eTimerCounterValue"
  Postion and Speed Calculation/2(theta) -> theta/1
  Postion and Speed Calculation/1("SpeedAct ") -> SpeedAct/1
  CurrentState/1 -> Postion and Speed Calculation/2(CurrentState)

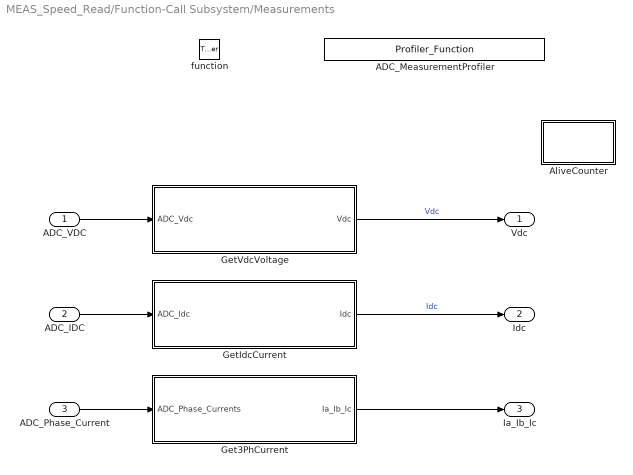
== system MEAS_Speed_Read/Function-Call Subsystem/Measurements ==
  ADC_VDC : Inport
  ADC_IDC : Inport  Port=2
  ADC_Phase_Current : Inport  Port=3
  function : TriggerPort  TriggerType=function-call  VariantControl=(inherit)
  ADC_MeasurementProfiler : mbd_mpc574x_ec_toolbox/Utility Blocks/Profiler_Function  profile_index=3
  AliveCounter : Subsystem
  Get3PhCurrent : Subsystem  Priority=1  TreatAsAtomicUnit=on
  GetIdcCurrent : Subsystem  Priority=3  TreatAsAtomicUnit=on
      settings: RTWFcnNameOpts=Use subsystem name
  GetVdcVoltage : Subsystem  Priority=2  TreatAsAtomicUnit=on
      settings: RTWFcnNameOpts=Use subsystem name
  Vdc : Outport
  Idc : Outport  Port=2
  Ia_Ib_Ic : Outport  Port=3
  wires:
  Get3PhCurrent/1(Ia_Ib_Ic) -> Ia_Ib_Ic/1
  ADC_Phase_Current/1 -> Get3PhCurrent/1(ADC_Phase_Currents)
  ADC_IDC/1 -> GetIdcCurrent/1(ADC_Idc)
  GetVdcVoltage/1(Vdc) -> Vdc/1  "Vdc"
  GetIdcCurrent/1(Idc) -> Idc/1  "Idc"
  ADC_VDC/1 -> GetVdcVoltage/1(ADC_Vdc)

== system MEAS_Speed_Read/Subsystem/Normalization on 2pi ==
  eTimerCounterValue : Inport
  Data Type Conversion1 : DataTypeConversion  OutDataTypeStr=single  SaturateOnIntegerOverflow=off  RndMeth=Floor
  Gain1 : Gain  Gain=2*pi/4000
  Theta0To2pi : Outport
  wires:
  eTimerCounterValue/1 -> Data Type Conversion1/1
  Gain1/1 -> Theta0To2pi/1
  Data Type Conversion1/1 -> Gain1/1

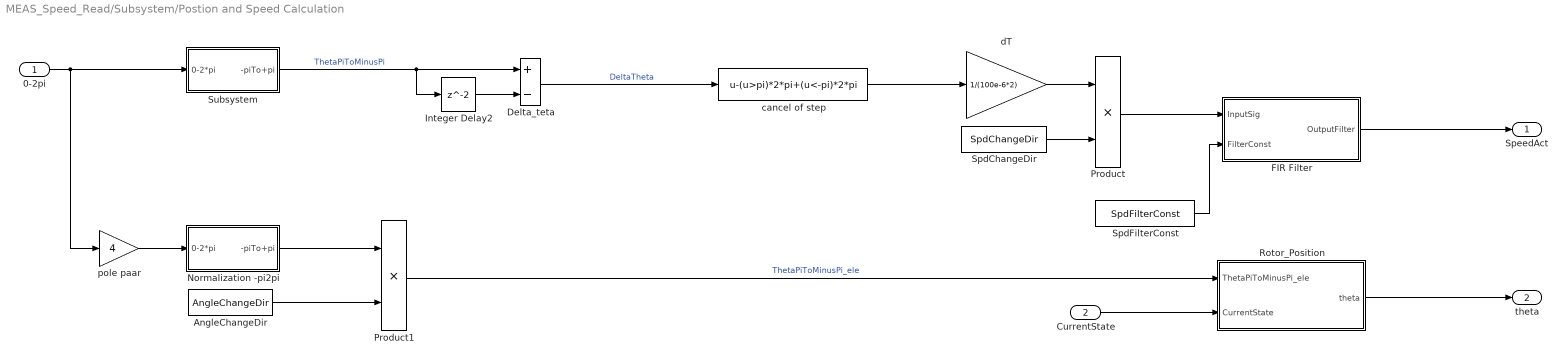
== system MEAS_Speed_Read/Subsystem/Postion and Speed Calculation ==
  0-2pi : Inport
  CurrentState : Inport  Port=2
  AngleChangeDir : Constant  Value=AngleChangeDir
  Delta_teta : Sum  Inputs=+-  InputSameDT=on  SaturateOnIntegerOverflow=on  OutDataTypeStr=Inherit: Same as first input
  FIR Filter : Subsystem
  Integer Delay2 : Delay
  Normalization -pi2pi : Subsystem
  Product : Product
  Product1 : Product
  Rotor_Position : Subsystem
  SpdChangeDir : Constant  Value=SpdChangeDir
  SpdFilterConst : Constant  Value=SpdFilterConst
  Subsystem : Subsystem
  cancel of step : Fcn  Expr=u-(u>pi)*2*pi+(u<-pi)*2*pi
  dT : Gain  Gain=1/(100e-6*2)  SaturateOnIntegerOverflow=on  OutDataTypeStr=Inherit: Same as input  ParamDataTypeStr=Inherit: Same as input
  pole paar : Gain  Gain=4  SaturateOnIntegerOverflow=on  OutDataTypeStr=Inherit: Same as input  ParamDataTypeStr=Inherit: Same as input
  "SpeedAct " : Outport
  theta : Outport  Port=2
  wires:
  Normalization -pi2pi/1(-piTo+pi) -> Product1/1
  AngleChangeDir/1 -> Product1/2
  Product1/1 -> Rotor_Position/1(ThetaPiToMinusPi_ele)  "ThetaPiToMinusPi_ele"
  pole paar/1 -> Normalization -pi2pi/1(0-2*pi)
  SpdFilterConst/1 -> FIR Filter/2(FilterConst)
  Product/1 -> FIR Filter/1(InputSig)
  SpdChangeDir/1 -> Product/2
  0-2pi/1 -> pole paar/1, Subsystem/1(0-2*pi)
  Subsystem/1(-piTo+pi) -> Delta_teta/1, Integer Delay2/1  "ThetaPiToMinusPi"
  cancel of step/1 -> dT/1
  FIR Filter/1(OutputFilter) -> "SpeedAct "/1
  Integer Delay2/1 -> Delta_teta/2
  dT/1 -> Product/1
  Delta_teta/1 -> cancel of step/1  "DeltaTheta"
  Rotor_Position/1(theta) -> theta/1
  CurrentState/1 -> Rotor_Position/2(CurrentState)

== system MEAS_Speed_Read/Function-Call Subsystem/Measurements/AliveCounter ==
  Constant : Constant
  Sum1 : Sum
  Unit Delay : UnitDelay  SampleTime=-1  HasFrameUpgradeWarning=on
  wires:
  Constant/1 -> Sum1/1
  Sum1/1 -> Unit Delay/1  "AliveCounterMeasurement"
  Unit Delay/1 -> Sum1/2

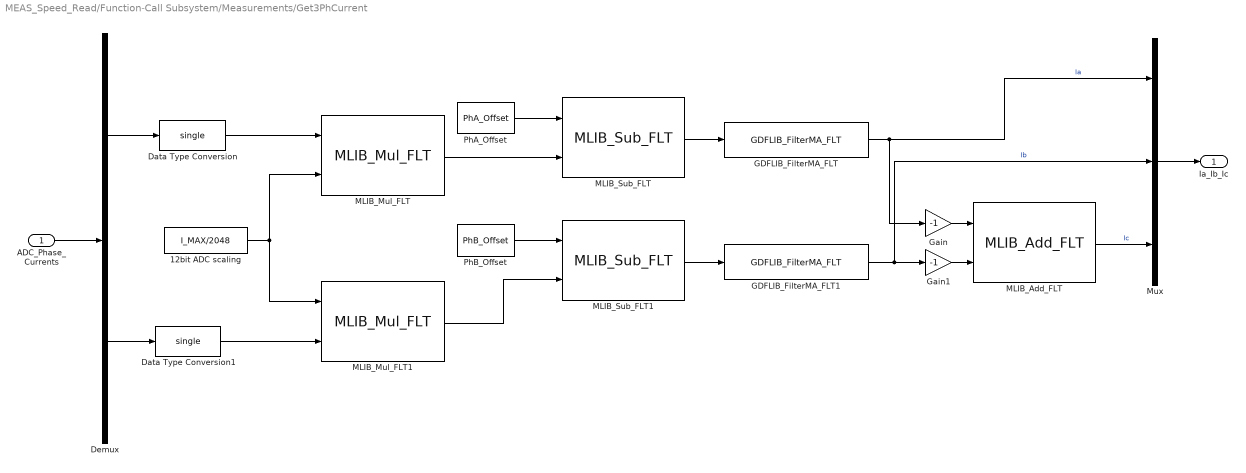
== system MEAS_Speed_Read/Function-Call Subsystem/Measurements/Get3PhCurrent ==
  ADC_Phase_Currents : Inport
  12bit ADC scaling : Constant  Value=I_MAX/2048  OutDataTypeStr=single
  Data Type Conversion : DataTypeConversion  OutDataTypeStr=single  SaturateOnIntegerOverflow=off  RndMeth=Floor
  Data Type Conversion1 : DataTypeConversion  OutDataTypeStr=single  SaturateOnIntegerOverflow=off  RndMeth=Floor
  Demux : Demux  Outputs=2
  GDFLIB_FilterMA_FLT : ammclib_bam_mpc574x/GDFLIB/bam_flt/GDFLIB_FilterMA_FLT  fltLambda=1/10
  GDFLIB_FilterMA_FLT1 : ammclib_bam_mpc574x/GDFLIB/bam_flt/GDFLIB_FilterMA_FLT  fltLambda=1/10
  Gain : Gain  Gain=-1  OutDataTypeStr=single
  Gain1 : Gain  Gain=-1  OutDataTypeStr=single
  MLIB_Add_FLT : ammclib_bam_mpc574x/MLIB/bam_flt/MLIB_Add_FLT
  MLIB_Mul_FLT : ammclib_bam_mpc574x/MLIB/bam_flt/MLIB_Mul_FLT
  MLIB_Mul_FLT1 : ammclib_bam_mpc574x/MLIB/bam_flt/MLIB_Mul_FLT
  MLIB_Sub_FLT : ammclib_bam_mpc574x/MLIB/bam_flt/MLIB_Sub_FLT
  MLIB_Sub_FLT1 : ammclib_bam_mpc574x/MLIB/bam_flt/MLIB_Sub_FLT
  Mux : Mux  Inputs=3
  PhA_Offset : Constant  Value=PhA_Offset  OutDataTypeStr=single
  PhB_Offset : Constant  Value=PhB_Offset  OutDataTypeStr=single
  Ia_Ib_Ic : Outport
  wires:
  GDFLIB_FilterMA_FLT1/1 -> Gain1/1, Mux/2  "Ib"
  MLIB_Sub_FLT1/1 -> GDFLIB_FilterMA_FLT1/1
  GDFLIB_FilterMA_FLT/1 -> Mux/1, Gain/1  "Ia"
  MLIB_Sub_FLT/1 -> GDFLIB_FilterMA_FLT/1
  MLIB_Add_FLT/1 -> Mux/3  "Ic"
  Demux/1 -> Data Type Conversion/1
  Demux/2 -> Data Type Conversion1/1
  Gain/1 -> MLIB_Add_FLT/1
  12bit ADC scaling/1 -> MLIB_Mul_FLT1/1, MLIB_Mul_FLT/2
  PhA_Offset/1 -> MLIB_Sub_FLT/1
  Data Type Conversion1/1 -> MLIB_Mul_FLT1/2
  Data Type Conversion/1 -> MLIB_Mul_FLT/1
  Gain1/1 -> MLIB_Add_FLT/2
  PhB_Offset/1 -> MLIB_Sub_FLT1/1
  MLIB_Mul_FLT/1 -> MLIB_Sub_FLT/2
  MLIB_Mul_FLT1/1 -> MLIB_Sub_FLT1/2
  ADC_Phase_Currents/1 -> Demux/1
  Mux/1 -> Ia_Ib_Ic/1

== system MEAS_Speed_Read/Function-Call Subsystem/Measurements/GetIdcCurrent ==
  ADC_Idc : Inport
  ADC_PB8 Offset and Logic power supply compensation : Constant  Value=2060  OutDataTypeStr=uint16
  MLIB_Mul_FLT : ammclib_bam_mpc574x/MLIB/bam_flt/MLIB_Mul_FLT
  Sum : Sum  Inputs=+-  OutDataTypeStr=single
  bits2amps : Constant  Value=16.5/2048  OutDataTypeStr=single
  Idc : Outport
  wires:
  MLIB_Mul_FLT/1 -> Idc/1
  Sum/1 -> MLIB_Mul_FLT/1
  ADC_PB8 Offset and Logic power supply compensation/1 -> Sum/2
  ADC_Idc/1 -> Sum/1
  bits2amps/1 -> MLIB_Mul_FLT/2

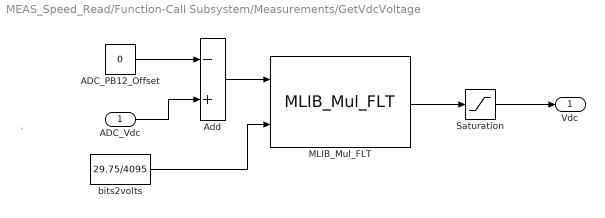
== system MEAS_Speed_Read/Function-Call Subsystem/Measurements/GetVdcVoltage ==
  note: `
  ADC_Vdc : Inport
  ADC_PB12_Offset : Constant  Value=0  OutDataTypeStr=uint16
  Add : Sum  Inputs=-+  InputSameDT=on  OutDataTypeStr=Inherit: Inherit via back propagation
  MLIB_Mul_FLT : ammclib_bam_mpc574x/MLIB/bam_flt/MLIB_Mul_FLT
  Saturation : Saturate  UpperLimit=29.75  LowerLimit=0
  bits2volts : Constant  Value=29.75/4095  OutDataTypeStr=single
  Vdc : Outport
  wires:
  Saturation/1 -> Vdc/1
  MLIB_Mul_FLT/1 -> Saturation/1
  Add/1 -> MLIB_Mul_FLT/1
  bits2volts/1 -> MLIB_Mul_FLT/2
  ADC_Vdc/1 -> Add/2
  ADC_PB12_Offset/1 -> Add/1

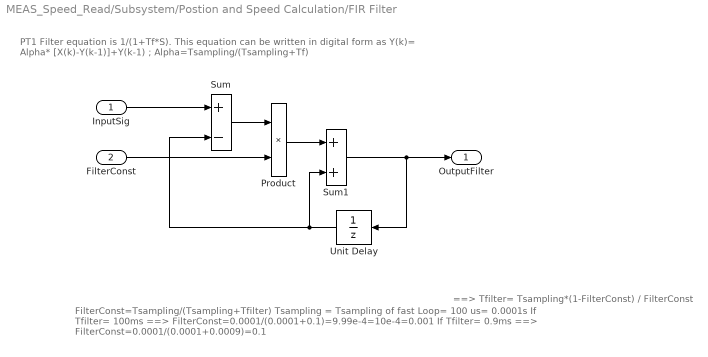
== system MEAS_Speed_Read/Subsystem/Postion and Speed Calculation/FIR Filter ==
  note: FilterConst=Tsampling/(Tsampling+Tfilter)
      | Tsampling = Tsampling of fast Loop= 100 us= 0.0001s
      |
      | If Tfilter= 100ms ==> FilterConst=0.0001/(0.0001+0.1)=9.99e-4=10e-4=0.001
      |
      | If Tfilter= 0.9ms ==> FilterConst=0.0001/(0.0001+0.0009)=0.1
  note: PT1 Filter equation is 1/(1+Tf*S). This equation can be written in digital form as
      | Y(k)= Alpha* [X(k)-Y(k-1)]+Y(k-1)
      | ; Alpha=Tsampling/(Tsampling+Tf)
  note: ==> Tfilter= Tsampling*(1-FilterConst) / FilterConst
  InputSig : Inport
  FilterConst : Inport  Port=2
  Product : Product
  Sum : Sum  Inputs=+-
  Sum1 : Sum
  Unit Delay : UnitDelay  SampleTime=-1  HasFrameUpgradeWarning=on
  OutputFilter : Outport
  wires:
  InputSig/1 -> Sum/1
  Sum1/1 -> Unit Delay/1, OutputFilter/1
  Product/1 -> Sum1/1
  FilterConst/1 -> Product/2
  Unit Delay/1 -> Sum1/2, Sum/2
  Sum/1 -> Product/1

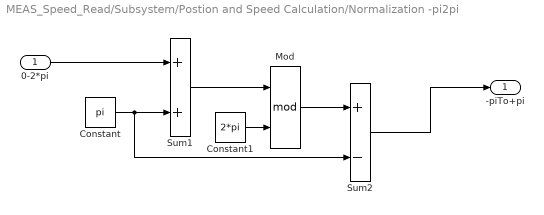
== system MEAS_Speed_Read/Subsystem/Postion and Speed Calculation/Normalization -pi2pi ==
  0-2*pi : Inport
  Constant : Constant  Value=pi  OutDataTypeStr=single
  Constant1 : Constant  Value=2*pi  OutDataTypeStr=single
  Mod : Math  Operator=mod
  Sum1 : Sum
  Sum2 : Sum  Inputs=+-
  -piTo+pi : Outport
  wires:
  Sum1/1 -> Mod/1
  Constant1/1 -> Mod/2
  Mod/1 -> Sum2/1
  Constant/1 -> Sum1/2, Sum2/2
  0-2*pi/1 -> Sum1/1
  Sum2/1 -> -piTo+pi/1

== system MEAS_Speed_Read/Subsystem/Postion and Speed Calculation/Rotor_Position ==
  note: ExecuteAlign = 1, During the alignment
      | ExecuteAlign = 0, After the alignment
      | ==> THETA will be 0 during the alignment
  ThetaPiToMinusPi_ele : Inport
  CurrentState : Inport  Port=2
  Align vs. Normal Operation : Switch  Threshold=2  SaturateOnIntegerOverflow=off  InputSameDT=off
  OffsetCalcn : Subsystem
  Standstill : Constant  Value=0  OutDataTypeStr=single  SampleTime=-1
  theta : Outport  OutDataTypeStr=single
  wires:
  OffsetCalcn/1(ThetaMeasWithOffsetNorm) -> Align vs. Normal Operation/1
  ThetaPiToMinusPi_ele/1 -> OffsetCalcn/1(ThetaPiToMinusPi_ele)
  Align vs. Normal Operation/1 -> theta/1
  Standstill/1 -> Align vs. Normal Operation/3
  CurrentState/1 -> OffsetCalcn/2(CurrentState), Align vs. Normal Operation/2

== system MEAS_Speed_Read/Subsystem/Postion and Speed Calculation/Subsystem ==
  0-2*pi : Inport
  Constant : Constant  Value=pi  OutDataTypeStr=single
  Sum2 : Sum  Inputs=+-
  -piTo+pi : Outport
  wires:
  Sum2/1 -> -piTo+pi/1
  0-2*pi/1 -> Sum2/1
  Constant/1 -> Sum2/2

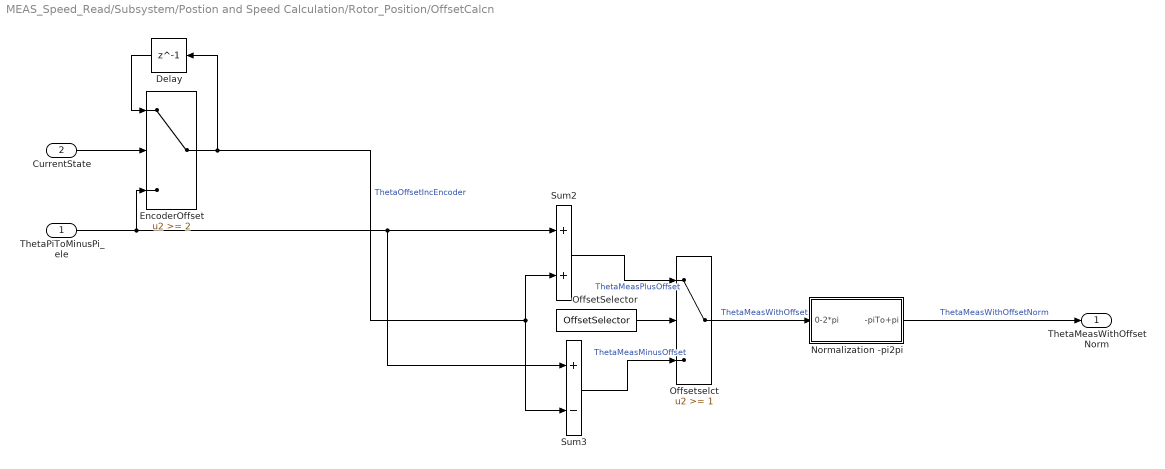
== system MEAS_Speed_Read/Subsystem/Postion and Speed Calculation/Rotor_Position/OffsetCalcn ==
  ThetaPiToMinusPi_ele : Inport
  CurrentState : Inport  Port=2
  Delay : Delay  DelayLength=1
  EncoderOffset : Switch  Threshold=2  SaturateOnIntegerOverflow=off  InputSameDT=off
  Normalization -pi2pi : Subsystem
  OffsetSelector : Constant  Value=OffsetSelector
  Offsetselct : Switch  Threshold=1  SaturateOnIntegerOverflow=off  InputSameDT=off
  Sum2 : Sum
  Sum3 : Sum  Inputs=+-
  ThetaMeasWithOffsetNorm : Outport
  wires:
  Normalization -pi2pi/1(-piTo+pi) -> ThetaMeasWithOffsetNorm/1  "ThetaMeasWithOffsetNorm"
  Offsetselct/1 -> Normalization -pi2pi/1(0-2*pi)  "ThetaMeasWithOffset"
  EncoderOffset/1 -> Sum3/2, Sum2/2, Delay/1  "ThetaOffsetIncEncoder"
  Sum3/1 -> Offsetselct/3  "ThetaMeasMinusOffset"
  OffsetSelector/1 -> Offsetselct/2
  ThetaPiToMinusPi_ele/1 -> EncoderOffset/3, Sum2/1, Sum3/1
  Sum2/1 -> Offsetselct/1  "ThetaMeasPlusOffset"
  Delay/1 -> EncoderOffset/1
  CurrentState/1 -> EncoderOffset/2

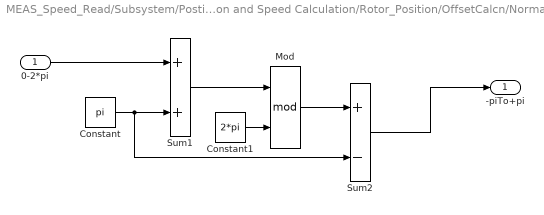
== system MEAS_Speed_Read/Subsystem/Postion and Speed Calculation/Rotor_Position/OffsetCalcn/Normalization -pi2pi ==
  0-2*pi : Inport
  Constant : Constant  Value=pi  OutDataTypeStr=single
  Constant1 : Constant  Value=2*pi  OutDataTypeStr=single
  Mod : Math  Operator=mod
  Sum1 : Sum
  Sum2 : Sum  Inputs=+-
  -piTo+pi : Outport
  wires:
  Sum1/1 -> Mod/1
  Constant1/1 -> Mod/2
  Mod/1 -> Sum2/1
  Constant/1 -> Sum1/2, Sum2/2
  0-2*pi/1 -> Sum1/1
  Sum2/1 -> -piTo+pi/1
